simulink model "fir"  (R2020a)
settings: Solver=FixedStepAuto  StartTime=0.0  StopTime=20  RelTol=1e-3
settings Model: Creator=sadamu  LastModifiedBy=sadamu
settings SolverCC: AutoInsertRateTranBlk=on
settings DataIOCC: LimitDataPoints=on  SaveOutput=off  SignalLogging=off  DSMLogging=off  SaveTime=off
settings OptimizationCC: DefaultParameterBehavior=Inlined  DefaultUnderspecifiedDataType=single  StrengthReduction=on  PassReuseOutputArgsAs=Individual arguments  ZeroExternalMemoryAtStartup=off  ZeroInternalMemoryAtStartup=off  OptimizeBlockOrder=speed  OptimizationPriority=Speed  OptimizationCustomize=off  MultiThreadedLoops=on  EfficientTunableParamExpr=on
settings DebuggingCC: AlgebraicLoopMsg=error  SingleTaskRateTransMsg=error  ParameterTunabilityLossMsg=error  AllowSymbolicDim=off  SFUnexpectedBacktrackingDiag=warning  SFNoUnconditionalDefaultTransitionDiag=warning  SFExecutionAtInitializationDiag=none  ArithmeticOperatorsInVariantConditions=warning
settings HardwareCC: ProdBitPerPointer=32  ProdBitPerSizeT=32  ProdBitPerPtrDiffT=32  ProdLargestAtomicInteger=Long  ProdLargestAtomicFloat=Double  ProdWordSize=32  ProdHWDeviceType=ARM Compatible->ARM Cortex
settings SFSimCC: SimUseLocalCustomCode=off  MATLABDynamicMemAlloc=off  CustomCodeUndefinedFunction=UseInterfaceOnly
settings RTWCC: SystemTargetFile=ert.tlc  GenCodeOnly=on  TemplateMakefile=ert_default_tmf  GenerateReport=on  RTWUseLocalCustomCode=off  BuildConfiguration=Debug  LaunchReport=on
settings CodeAppCC: GenerateComments=off  IgnoreCustomStorageClasses=off  OperatorAnnotations=on  SimulinkDataObjDesc=on  SFDataObjDesc=on  InsertBlockDesc=on  EnableCustomComments=on
settings ERTTargetCC: CodeReplacementLibrary=Inlined ARM NEON Intrinsics  GenerateSampleERTMain=on  InlinedParameterPlacement=NonHierarchical  ERTCustomFileTemplate=example_file_process.tlc

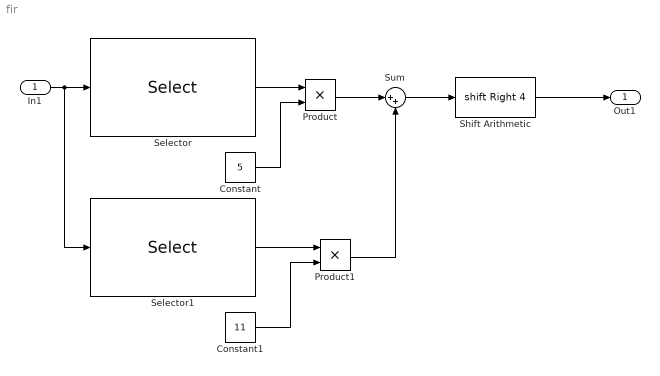
== system fir ==
  In1 : Inport  OutDataTypeStr=int32  PortDimensions=1025
  Constant : Constant  Value=5  OutDataTypeStr=int32
  Constant1 : Constant  Value=11  OutDataTypeStr=int32
  Product : Product  OutDataTypeStr=int32
  Product1 : Product  OutDataTypeStr=int32
  Selector : Selector  InputPortWidth=1025  IndexOptions=Starting index (dialog)  Indices=[1]  OutputSizes=1024
  Selector1 : Selector  InputPortWidth=1025  IndexOptions=Starting index (dialog)  Indices=[2]  OutputSizes=1024
  Shift Arithmetic : ArithShift  BitShiftNumber=4  BitShiftDirection=Right
  Sum : Sum  Inputs=|++  OutDataTypeStr=Inherit: Inherit via back propagation
  Out1 : Outport
  wires:
  Selector1/1 -> Product1/1
  In1/1 -> Selector1/1, Selector/1
  Constant/1 -> Product/2
  Selector/1 -> Product/1
  Product1/1 -> Sum/2
  Product/1 -> Sum/1
  Sum/1 -> Shift Arithmetic/1
  Constant1/1 -> Product1/2
  Shift Arithmetic/1 -> Out1/1
